simulink model "GNC_functional_diagram"  (R2021b)
settings: Solver=VariableStepAuto  StartTime=0.0  StopTime=10.0  RelTol=1e-3
model workspace (MAT data in the model file):
  AV_Status_Signal = Simulink.Bus
  AV_Status_Signal.Alignment = -1
  AV_Status_Signal.PreserveElementDimensions = 0
  AV_Status_Signal.Elements_internal(1) = Simulink.BusElement
  AV_Status_Signal.Elements_internal(1).DimensionsMode = 'Fixed'
  AV_Status_Signal.Elements_internal(1).SamplingMode = 'Sample based'
  AV_Status_Signal.Elements_internal(1).SampleTime = -1
  AV_Status_Signal.Elements_internal(1).Name = 'Detumbling_Trigger'
  AV_Status_Signal.Elements_internal(1).DataType_internal = 'double'
  AV_Status_Signal.Elements_internal(1).Complexity = 'real'
  AV_Status_Signal.Elements_internal(1).Dimensions = 1
  AV_Status_Signal.Elements_internal(2) = Simulink.BusElement
  AV_Status_Signal.Elements_internal(2).DimensionsMode = 'Fixed'
  AV_Status_Signal.Elements_internal(2).SamplingMode = 'Sample based'
  AV_Status_Signal.Elements_internal(2).SampleTime = -1
  AV_Status_Signal.Elements_internal(2).Name = 'Testing_Trigger'
  AV_Status_Signal.Elements_internal(2).DataType_internal = 'double'
  AV_Status_Signal.Elements_internal(2).Complexity = 'real'
  AV_Status_Signal.Elements_internal(2).Dimensions = 1
  AV_Status_Signal.DataScope = 'Auto'
  Resources_Budget = Simulink.Bus
  Resources_Budget.Alignment = -1
  Resources_Budget.PreserveElementDimensions = 0
  Resources_Budget.Elements_internal(1) = Simulink.BusElement
  Resources_Budget.Elements_internal(1).DimensionsMode = 'Fixed'
  Resources_Budget.Elements_internal(1).SamplingMode = 'Sample based'
  Resources_Budget.Elements_internal(1).SampleTime = -1
  Resources_Budget.Elements_internal(1).Name = 'Processing_Power'
  Resources_Budget.Elements_internal(1).DataType_internal = 'double'
  Resources_Budget.Elements_internal(1).Complexity = 'real'
  Resources_Budget.Elements_internal(1).Dimensions = 1
  Resources_Budget.Elements_internal(2) = Simulink.BusElement
  Resources_Budget.Elements_internal(2).DimensionsMode = 'Fixed'
  Resources_Budget.Elements_internal(2).SamplingMode = 'Sample based'
  Resources_Budget.Elements_internal(2).SampleTime = -1
  Resources_Budget.Elements_internal(2).Name = 'Memory_Allocation'
  Resources_Budget.Elements_internal(2).DataType_internal = 'double'
  Resources_Budget.Elements_internal(2).Complexity = 'real'
  Resources_Budget.Elements_internal(2).Dimensions = 1
  Resources_Budget.Elements_internal(3) = Simulink.BusElement
  Resources_Budget.Elements_internal(3).DimensionsMode = 'Fixed'
  Resources_Budget.Elements_internal(3).SamplingMode = 'Sample based'
  Resources_Budget.Elements_internal(3).SampleTime = -1
  Resources_Budget.Elements_internal(3).Name = 'Power'
  Resources_Budget.Elements_internal(3).DataType_internal = 'double'
  Resources_Budget.Elements_internal(3).Complexity = 'real'
  Resources_Budget.Elements_internal(3).Dimensions = 1
  Resources_Budget.DataScope = 'Auto'
  Sensor_Signal = Simulink.Bus
  Sensor_Signal.Alignment = -1
  Sensor_Signal.PreserveElementDimensions = 0
  Sensor_Signal.Elements_internal(1) = Simulink.BusElement
  Sensor_Signal.Elements_internal(1).DimensionsMode = 'Fixed'
  Sensor_Signal.Elements_internal(1).SamplingMode = 'Sample based'
  Sensor_Signal.Elements_internal(1).SampleTime = -1
  Sensor_Signal.Elements_internal(1).Name = 'Sun_Sensor_Measurment'
  Sensor_Signal.Elements_internal(1).DataType_internal = 'double'
  Sensor_Signal.Elements_internal(1).Complexity = 'real'
  Sensor_Signal.Elements_internal(1).Dimensions = 1
  Sensor_Signal.Elements_internal(2) = Simulink.BusElement
  Sensor_Signal.Elements_internal(2).DimensionsMode = 'Fixed'
  Sensor_Signal.Elements_internal(2).SamplingMode = 'Sample based'
  Sensor_Signal.Elements_internal(2).SampleTime = -1
  Sensor_Signal.Elements_internal(2).Name = 'IMU_Measurement'
  Sensor_Signal.Elements_internal(2).DataType_internal = 'double'
  Sensor_Signal.Elements_internal(2).Complexity = 'real'
  Sensor_Signal.Elements_internal(2).Dimensions = 1
  Sensor_Signal.DataScope = 'Auto'
settings Model: Creator=jonas  LastModifiedBy=leoba

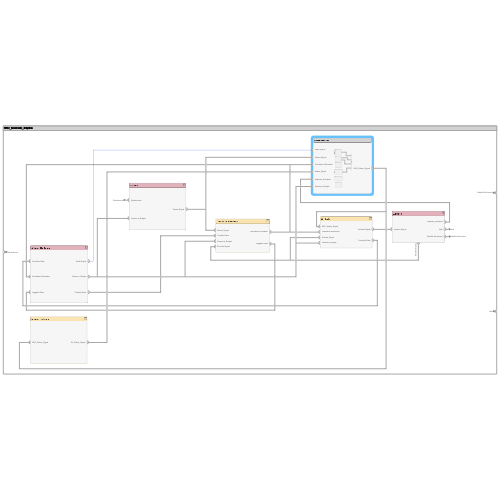
[thumbnail: Simulink's stored preview of the top-level diagram]
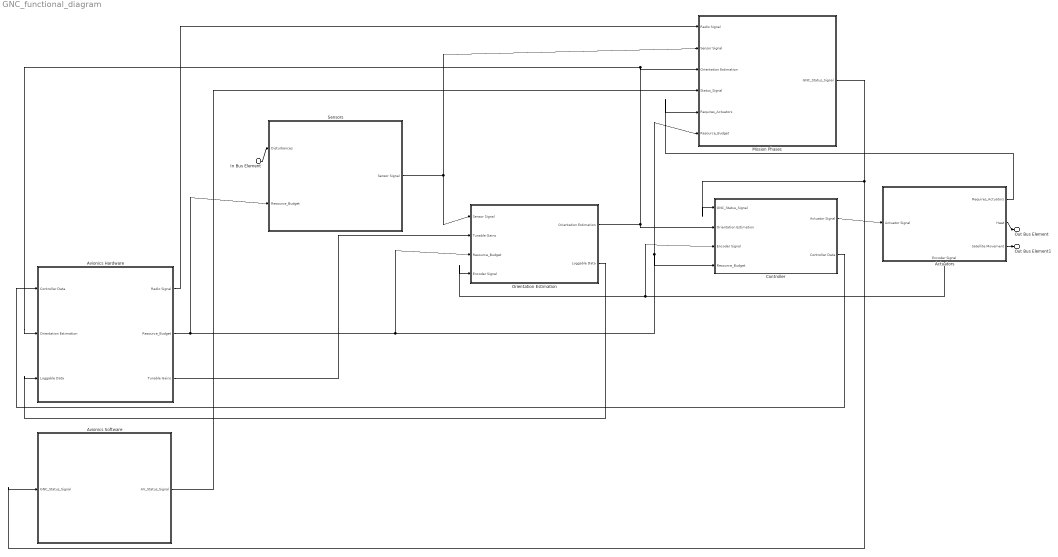
== system GNC_functional_diagram ==
  In Bus Element : Inport  PortName=Disturbances
  Actuators : Subsystem
      settings: PortSchema="{\"entries\":[{\"content\":{\"headerSize\":26,\"margin\":15,\"minimumSpacing\":25,\"sides\":[{\"content\":{\"connectorIds\":[\"In1\"]},\"type\":\"ConnectorPlacement.EquallySpacedRectSide\",\"uuid\":\"4d219d8c-999e-4fa6-ade9-cc6ac14ded32\"},{\"content\":{\"connectorIds\":[\"Out1\",\"Out2\",\"Out3\"],\"side\":\"RIGHT\"},\"type\":\"ConnectorPlacement.EquallySpacedRectSide\",\"uuid\":\"291554bf-cd30-4ae6-93e5-4052e0d4037d\"},{\"content\":{\"connectorIds\":[],\"side\":\"TOP\"},\"type\":\"ConnectorPlacement.EquallySpacedRectSide\",\"uuid\":\"a407b5ba-b8ce-49a8-af7c-64b4689399b6\"},{\"content\":{\"connectorIds\":[\"Out4\"],\"side\":\"BOTTOM\"},\"type\":\"ConnectorPlacement.EquallySpacedRectSide\",\"uuid\":\"28acc806-9e86-4bc6-af71-2b4411156648\"}]},\"type\":\"ConnectorPlacement.EquallySpacedConnector\",\"uuid\":\"1a65b071-c199-4364-8343-b80f4df9252b\"}],\"packageUris\":[\"http://schema.mathworks.com/mf0/Connector/R2020b\"],\"version\":\"1.0\"}"
  Avionics Hardware : Subsystem
      settings: PortSchema="{\"entries\":[{\"content\":{\"headerSize\":26,\"margin\":15,\"minimumSpacing\":25,\"sides\":[{\"content\":{\"connectorIds\":[\"In1\",\"In3\",\"In2\"]},\"type\":\"ConnectorPlacement.EquallySpacedRectSide\",\"uuid\":\"4d219d8c-999e-4fa6-ade9-cc6ac14ded32\"},{\"content\":{\"connectorIds\":[\"Out1\",\"Out2\",\"Out3\"],\"side\":\"RIGHT\"},\"type\":\"ConnectorPlacement.EquallySpacedRectSide\",\"uuid\":\"291554bf-cd30-4ae6-93e5-4052e0d4037d\"},{\"content\":{\"connectorIds\":[],\"side\":\"TOP\"},\"type\":\"ConnectorPlacement.EquallySpacedRectSide\",\"uuid\":\"a407b5ba-b8ce-49a8-af7c-64b4689399b6\"},{\"content\":{\"connectorIds\":[],\"side\":\"BOTTOM\"},\"type\":\"ConnectorPlacement.EquallySpacedRectSide\",\"uuid\":\"eed5de48-d554-4a4a-aaed-8ac1beb8b61e\"}]},\"type\":\"ConnectorPlacement.EquallySpacedConnector\",\"uuid\":\"1a65b071-c199-4364-8343-b80f4df9252b\"}],\"packageUris\":[\"http://schema.mathworks.com/mf0/Connector/R2020b\"],\"version\":\"1.0\"}"
  Avionics Software : Subsystem
      settings: PortSchema="{\"entries\":[{\"content\":{\"headerSize\":26,\"margin\":15,\"minimumSpacing\":25,\"sides\":[{\"content\":{\"connectorIds\":[\"In1\"]},\"type\":\"ConnectorPlacement.EquallySpacedRectSide\",\"uuid\":\"9c9f921c-2c3b-482c-ae0a-30fa5cf19172\"},{\"content\":{\"connectorIds\":[\"Out1\"],\"side\":\"RIGHT\"},\"type\":\"ConnectorPlacement.EquallySpacedRectSide\",\"uuid\":\"566c4868-5865-4e1f-981e-d74a35c979c9\"},{\"content\":{\"connectorIds\":[],\"side\":\"TOP\"},\"type\":\"ConnectorPlacement.EquallySpacedRectSide\",\"uuid\":\"2cd88ae2-a2e5-4e25-b817-9d229c73c4c9\"}]},\"type\":\"ConnectorPlacement.EquallySpacedConnector\",\"uuid\":\"48eadbd9-1de4-4fec-af56-45dc4412e923\"}],\"packageUris\":[\"http://schema.mathworks.com/mf0/Connector/R2020b\"],\"version\":\"1.0\"}"
  Controller : Subsystem
      settings: PortSchema="{\"entries\":[{\"content\":{\"headerSize\":26,\"margin\":15,\"minimumSpacing\":25,\"sides\":[{\"content\":{\"connectorIds\":[\"In1\",\"In2\",\"In3\",\"In4\"]},\"type\":\"ConnectorPlacement.EquallySpacedRectSide\",\"uuid\":\"4d219d8c-999e-4fa6-ade9-cc6ac14ded32\"},{\"content\":{\"connectorIds\":[\"Out1\",\"Out2\"],\"side\":\"RIGHT\"},\"type\":\"ConnectorPlacement.EquallySpacedRectSide\",\"uuid\":\"291554bf-cd30-4ae6-93e5-4052e0d4037d\"},{\"content\":{\"connectorIds\":[],\"side\":\"TOP\"},\"type\":\"ConnectorPlacement.EquallySpacedRectSide\",\"uuid\":\"a407b5ba-b8ce-49a8-af7c-64b4689399b6\"}]},\"type\":\"ConnectorPlacement.EquallySpacedConnector\",\"uuid\":\"1a65b071-c199-4364-8343-b80f4df9252b\"}],\"packageUris\":[\"http://schema.mathworks.com/mf0/Connector/R2020b\"],\"version\":\"1.0\"}"
  Mission Phases : Subsystem
      settings: PortSchema="{\"entries\":[{\"content\":{\"headerSize\":26,\"margin\":15,\"minimumSpacing\":25,\"sides\":[{\"content\":{\"connectorIds\":[\"In1\",\"In2\",\"In3\",\"In4\",\"In5\",\"In6\"]},\"type\":\"ConnectorPlacement.EquallySpacedRectSide\",\"uuid\":\"9c9f921c-2c3b-482c-ae0a-30fa5cf19172\"},{\"content\":{\"connectorIds\":[\"Out1\"],\"side\":\"RIGHT\"},\"type\":\"ConnectorPlacement.EquallySpacedRectSide\",\"uuid\":\"566c4868-5865-4e1f-981e-d74a35c979c9\"},{\"content\":{\"connectorIds\":[],\"side\":\"TOP\"},\"type\":\"ConnectorPlacement.EquallySpacedRectSide\",\"uuid\":\"2cd88ae2-a2e5-4e25-b817-9d229c73c4c9\"}]},\"type\":\"ConnectorPlacement.EquallySpacedConnector\",\"uuid\":\"48eadbd9-1de4-4fec-af56-45dc4412e923\"}],\"packageUris\":[\"http://schema.mathworks.com/mf0/Connector/R2020b\"],\"version\":\"1.0\"}"
  Orientation Estimation : Subsystem
      settings: PortSchema="{\"entries\":[{\"content\":{\"headerSize\":26,\"margin\":15,\"minimumSpacing\":25,\"sides\":[{\"content\":{\"connectorIds\":[\"In1\",\"In2\",\"In3\",\"In4\"]},\"type\":\"ConnectorPlacement.EquallySpacedRectSide\",\"uuid\":\"4d219d8c-999e-4fa6-ade9-cc6ac14ded32\"},{\"content\":{\"connectorIds\":[\"Out1\",\"Out2\"],\"side\":\"RIGHT\"},\"type\":\"ConnectorPlacement.EquallySpacedRectSide\",\"uuid\":\"291554bf-cd30-4ae6-93e5-4052e0d4037d\"},{\"content\":{\"connectorIds\":[],\"side\":\"TOP\"},\"type\":\"ConnectorPlacement.EquallySpacedRectSide\",\"uuid\":\"a407b5ba-b8ce-49a8-af7c-64b4689399b6\"}]},\"type\":\"ConnectorPlacement.EquallySpacedConnector\",\"uuid\":\"1a65b071-c199-4364-8343-b80f4df9252b\"}],\"packageUris\":[\"http://schema.mathworks.com/mf0/Connector/R2020b\"],\"version\":\"1.0\"}"
  Sensors : Subsystem
      settings: PortSchema="{\"entries\":[{\"content\":{\"headerSize\":26,\"margin\":15,\"minimumSpacing\":25,\"sides\":[{\"content\":{\"connectorIds\":[\"In1\",\"In2\"]},\"type\":\"ConnectorPlacement.EquallySpacedRectSide\",\"uuid\":\"4d219d8c-999e-4fa6-ade9-cc6ac14ded32\"},{\"content\":{\"connectorIds\":[\"Out1\"],\"side\":\"RIGHT\"},\"type\":\"ConnectorPlacement.EquallySpacedRectSide\",\"uuid\":\"291554bf-cd30-4ae6-93e5-4052e0d4037d\"},{\"content\":{\"connectorIds\":[],\"side\":\"TOP\"},\"type\":\"ConnectorPlacement.EquallySpacedRectSide\",\"uuid\":\"a407b5ba-b8ce-49a8-af7c-64b4689399b6\"}]},\"type\":\"ConnectorPlacement.EquallySpacedConnector\",\"uuid\":\"1a65b071-c199-4364-8343-b80f4df9252b\"}],\"packageUris\":[\"http://schema.mathworks.com/mf0/Connector/R2020b\"],\"version\":\"1.0\"}"
  Out Bus Element1 : Outport  PortName=Satellite Movement
  Out Bus Element : Outport  Port=2  PortName=Heat
  wires:
  Orientation Estimation/1(Orientation Estimation) -> Avionics Hardware/3(Orientation Estimation), Mission Phases/3(Orientation Estimation), Controller/2(Orientation Estimation)
  Orientation Estimation/2(Loggable Data) -> Avionics Hardware/2(Loggable Data)
  Avionics Hardware/3(Tunable Gains) -> Orientation Estimation/2(Tunable Gains)
  Controller/1(Actuator Signal) -> Actuators/1(Actuator Signal)
  Controller/2(Controller Data) -> Avionics Hardware/1(Controller Data)
  Actuators/4(Encoder Signal) -> Orientation Estimation/4(Encoder Signal), Controller/3(Encoder Signal)
  Actuators/2(Heat) -> Out Bus Element/1
  Actuators/3(Satellite Movement) -> Out Bus Element1/1
  In Bus Element/1 -> Sensors/1(Disturbances)
  Avionics Hardware/1(Radio Signal) -> Mission Phases/1(Radio Signal)
  Sensors/1(Sensor Signal) -> Mission Phases/2(Sensor Signal), Orientation Estimation/1(Sensor Signal)
  Avionics Software/1(AV_Status_Signal) -> Mission Phases/4(Status_Signal)
  Actuators/1(Requires_Actuators) -> Mission Phases/5(Requires_Actuators)
  Mission Phases/1(GNC_Status_Signal) -> Controller/1(GNC_Status_Signal), Avionics Software/1(GNC_Status_Signal)
  Avionics Hardware/2(Resource_Budget) -> Sensors/2(Resource_Budget), Controller/4(Resource_Budget), Mission Phases/6(Resource_Budget), Orientation Estimation/3(Resource_Budget)

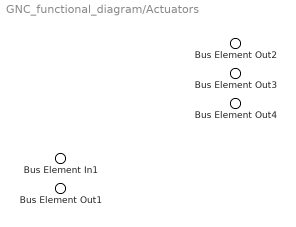
== system GNC_functional_diagram/Actuators ==
  Bus Element In1 : Inport  PortName=Actuator Signal
  Bus Element Out4 : Outport  PortName=Requires_Actuators
  Bus Element Out2 : Outport  Port=2  PortName=Heat
  Bus Element Out3 : Outport  Port=3  PortName=Satellite Movement
  Bus Element Out1 : Outport  Port=4  PortName=Encoder Signal

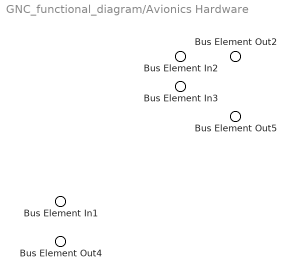
== system GNC_functional_diagram/Avionics Hardware ==
  Bus Element In3 : Inport  PortName=Controller Data
  Bus Element In2 : Inport  Port=2  PortName=Loggable Data
  Bus Element In1 : Inport  Port=3  PortName=Orientation Estimation
  Bus Element Out5 : Outport  PortName=Radio Signal
  Bus Element Out2 : Outport  Port=2  PortName=Resource_Budget
  Bus Element Out4 : Outport  Port=3  PortName=Tunable Gains

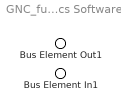
== system GNC_functional_diagram/Avionics Software ==
  Bus Element In1 : Inport  PortName=GNC_Status_Signal
  Bus Element Out1 : Outport  PortName=AV_Status_Signal

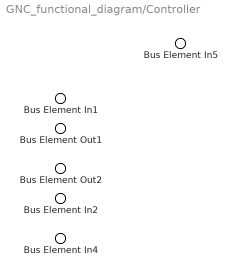
== system GNC_functional_diagram/Controller ==
  Bus Element In5 : Inport  PortName=GNC_Status_Signal
  Bus Element In1 : Inport  Port=2  PortName=Orientation Estimation
  Bus Element In2 : Inport  Port=3  PortName=Encoder Signal
  Bus Element In4 : Inport  Port=4  PortName=Resource_Budget
  Bus Element Out1 : Outport  PortName=Actuator Signal
  Bus Element Out2 : Outport  Port=2  PortName=Controller Data

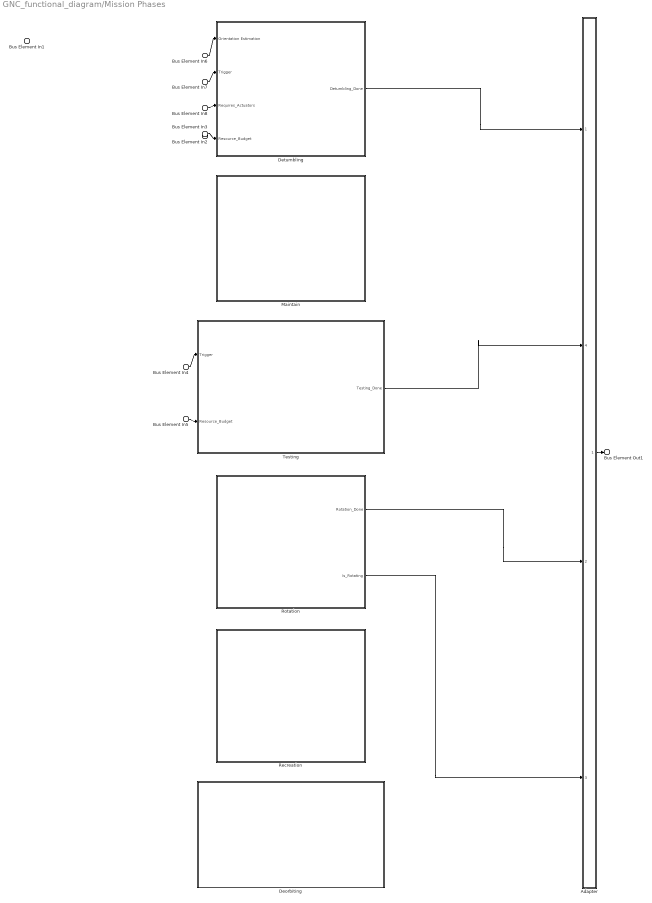
== system GNC_functional_diagram/Mission Phases ==
  Bus Element In1 : Inport  PortName=Radio Signal
  Bus Element In2 : Inport  Port=2  PortName=Sensor Signal
  Bus Element In6 : Inport  Port=3  PortName=Orientation Estimation
  Bus Element In7 : Inport  Port=4  PortName=Status_Signal  Element=Detumbling_Trigger
  Bus Element In4 : Inport  Port=4  PortName=Status_Signal  Element=Testing_Trigger
  Bus Element In8 : Inport  Port=5  PortName=Requires_Actuators
  Bus Element In3 : Inport  Port=6  PortName=Resource_Budget
  Bus Element In5 : Inport  Port=6  PortName=Resource_Budget
  Adapter : Subsystem
      settings: PortSchema="{\"entries\":[{\"content\":{\"margin\":10,\"minimumSpacing\":15,\"sides\":[{\"content\":{\"connectorIds\":[\"In1\",\"In4\",\"In2\",\"In3\"]},\"type\":\"ConnectorPlacement.EquallySpacedRectSide\",\"uuid\":\"9c9f921c-2c3b-482c-ae0a-30fa5cf19172\"},{\"content\":{\"connectorIds\":[\"Out1\"],\"side\":\"RIGHT\"},\"type\":\"ConnectorPlacement.EquallySpacedRectSide\",\"uuid\":\"566c4868-5865-4e1f-981e-d74a35c979c9\"},{\"content\":{\"connectorIds\":[],\"side\":\"TOP\"},\"type\":\"ConnectorPlacement.EquallySpacedRectSide\",\"uuid\":\"2cd88ae2-a2e5-4e25-b817-9d229c73c4c9\"}]},\"type\":\"ConnectorPlacement.EquallySpacedConnector\",\"uuid\":\"48eadbd9-1de4-4fec-af56-45dc4412e923\"}],\"packageUris\":[\"http://schema.mathworks.com/mf0/Connector/R2020b\"],\"version\":\"1.0\"}"
  Deorbiting : Subsystem
      settings: PortSchema="{\"entries\":[{\"content\":{\"headerSize\":26,\"margin\":15,\"minimumSpacing\":25,\"sides\":[{\"content\":{\"connectorIds\":[]},\"type\":\"ConnectorPlacement.EquallySpacedRectSide\",\"uuid\":\"9c9f921c-2c3b-482c-ae0a-30fa5cf19172\"},{\"content\":{\"connectorIds\":[],\"side\":\"RIGHT\"},\"type\":\"ConnectorPlacement.EquallySpacedRectSide\",\"uuid\":\"566c4868-5865-4e1f-981e-d74a35c979c9\"},{\"content\":{\"connectorIds\":[],\"side\":\"TOP\"},\"type\":\"ConnectorPlacement.EquallySpacedRectSide\",\"uuid\":\"2cd88ae2-a2e5-4e25-b817-9d229c73c4c9\"}]},\"type\":\"ConnectorPlacement.EquallySpacedConnector\",\"uuid\":\"48eadbd9-1de4-4fec-af56-45dc4412e923\"}],\"packageUris\":[\"http://schema.mathworks.com/mf0/Connector/R2020b\"],\"version\":\"1.0\"}"
  Detumbling : Subsystem
      settings: PortSchema="{\"entries\":[{\"content\":{\"headerSize\":26,\"margin\":15,\"minimumSpacing\":25,\"sides\":[{\"content\":{\"connectorIds\":[\"In1\",\"In2\",\"In3\",\"In4\"]},\"type\":\"ConnectorPlacement.EquallySpacedRectSide\",\"uuid\":\"9c9f921c-2c3b-482c-ae0a-30fa5cf19172\"},{\"content\":{\"connectorIds\":[\"Out1\"],\"side\":\"RIGHT\"},\"type\":\"ConnectorPlacement.EquallySpacedRectSide\",\"uuid\":\"566c4868-5865-4e1f-981e-d74a35c979c9\"},{\"content\":{\"connectorIds\":[],\"side\":\"TOP\"},\"type\":\"ConnectorPlacement.EquallySpacedRectSide\",\"uuid\":\"2cd88ae2-a2e5-4e25-b817-9d229c73c4c9\"}]},\"type\":\"ConnectorPlacement.EquallySpacedConnector\",\"uuid\":\"48eadbd9-1de4-4fec-af56-45dc4412e923\"}],\"packageUris\":[\"http://schema.mathworks.com/mf0/Connector/R2020b\"],\"version\":\"1.0\"}"
  Maintain : Subsystem
      settings: PortSchema="{\"entries\":[{\"content\":{\"headerSize\":26,\"margin\":15,\"minimumSpacing\":25,\"sides\":[{\"content\":{\"connectorIds\":[]},\"type\":\"ConnectorPlacement.EquallySpacedRectSide\",\"uuid\":\"9c9f921c-2c3b-482c-ae0a-30fa5cf19172\"},{\"content\":{\"connectorIds\":[],\"side\":\"RIGHT\"},\"type\":\"ConnectorPlacement.EquallySpacedRectSide\",\"uuid\":\"566c4868-5865-4e1f-981e-d74a35c979c9\"},{\"content\":{\"connectorIds\":[],\"side\":\"TOP\"},\"type\":\"ConnectorPlacement.EquallySpacedRectSide\",\"uuid\":\"2cd88ae2-a2e5-4e25-b817-9d229c73c4c9\"}]},\"type\":\"ConnectorPlacement.EquallySpacedConnector\",\"uuid\":\"48eadbd9-1de4-4fec-af56-45dc4412e923\"}],\"packageUris\":[\"http://schema.mathworks.com/mf0/Connector/R2020b\"],\"version\":\"1.0\"}"
  Recreation : Subsystem
      settings: PortSchema="{\"entries\":[{\"content\":{\"headerSize\":26,\"margin\":15,\"minimumSpacing\":25,\"sides\":[{\"content\":{\"connectorIds\":[]},\"type\":\"ConnectorPlacement.EquallySpacedRectSide\",\"uuid\":\"9c9f921c-2c3b-482c-ae0a-30fa5cf19172\"},{\"content\":{\"connectorIds\":[],\"side\":\"RIGHT\"},\"type\":\"ConnectorPlacement.EquallySpacedRectSide\",\"uuid\":\"566c4868-5865-4e1f-981e-d74a35c979c9\"},{\"content\":{\"connectorIds\":[],\"side\":\"TOP\"},\"type\":\"ConnectorPlacement.EquallySpacedRectSide\",\"uuid\":\"2cd88ae2-a2e5-4e25-b817-9d229c73c4c9\"}]},\"type\":\"ConnectorPlacement.EquallySpacedConnector\",\"uuid\":\"48eadbd9-1de4-4fec-af56-45dc4412e923\"}],\"packageUris\":[\"http://schema.mathworks.com/mf0/Connector/R2020b\"],\"version\":\"1.0\"}"
  Rotation : Subsystem
      settings: PortSchema="{\"entries\":[{\"content\":{\"headerSize\":26,\"margin\":15,\"minimumSpacing\":25,\"sides\":[{\"content\":{\"connectorIds\":[]},\"type\":\"ConnectorPlacement.EquallySpacedRectSide\",\"uuid\":\"9c9f921c-2c3b-482c-ae0a-30fa5cf19172\"},{\"content\":{\"connectorIds\":[\"Out1\",\"Out2\"],\"side\":\"RIGHT\"},\"type\":\"ConnectorPlacement.EquallySpacedRectSide\",\"uuid\":\"566c4868-5865-4e1f-981e-d74a35c979c9\"},{\"content\":{\"connectorIds\":[],\"side\":\"TOP\"},\"type\":\"ConnectorPlacement.EquallySpacedRectSide\",\"uuid\":\"2cd88ae2-a2e5-4e25-b817-9d229c73c4c9\"}]},\"type\":\"ConnectorPlacement.EquallySpacedConnector\",\"uuid\":\"48eadbd9-1de4-4fec-af56-45dc4412e923\"}],\"packageUris\":[\"http://schema.mathworks.com/mf0/Connector/R2020b\"],\"version\":\"1.0\"}"
  Testing : Subsystem
      settings: PortSchema="{\"entries\":[{\"content\":{\"headerSize\":26,\"margin\":15,\"minimumSpacing\":25,\"sides\":[{\"content\":{\"connectorIds\":[\"In1\",\"In2\"]},\"type\":\"ConnectorPlacement.EquallySpacedRectSide\",\"uuid\":\"9c9f921c-2c3b-482c-ae0a-30fa5cf19172\"},{\"content\":{\"connectorIds\":[\"Out1\"],\"side\":\"RIGHT\"},\"type\":\"ConnectorPlacement.EquallySpacedRectSide\",\"uuid\":\"566c4868-5865-4e1f-981e-d74a35c979c9\"},{\"content\":{\"connectorIds\":[],\"side\":\"TOP\"},\"type\":\"ConnectorPlacement.EquallySpacedRectSide\",\"uuid\":\"2cd88ae2-a2e5-4e25-b817-9d229c73c4c9\"}]},\"type\":\"ConnectorPlacement.EquallySpacedConnector\",\"uuid\":\"48eadbd9-1de4-4fec-af56-45dc4412e923\"}],\"packageUris\":[\"http://schema.mathworks.com/mf0/Connector/R2020b\"],\"version\":\"1.0\"}"
  Bus Element Out1 : Outport  PortName=GNC_Status_Signal
  wires:
  Bus Element In6/1 -> Detumbling/1(Orientation Estimation)
  Bus Element In7/1 -> Detumbling/2(Trigger)
  Bus Element In8/1 -> Detumbling/3(Requires_Actuators)
  Detumbling/1(Detumbling_Done) -> Adapter/1(Detumbling_Done)
  Rotation/1(Rotation_Done) -> Adapter/2(Rotation_Done)
  Rotation/2(Is_Rotating) -> Adapter/3(Is_Rotating)
  Adapter/1(GNC_Status_) -> Bus Element Out1/1
  Bus Element In3/1 -> Detumbling/4(Resource_Budget)
  Testing/1(Testing_Done) -> Adapter/4(Testing_Done)
  Bus Element In4/1 -> Testing/1(Trigger)
  Bus Element In5/1 -> Testing/2(Resource_Budget)

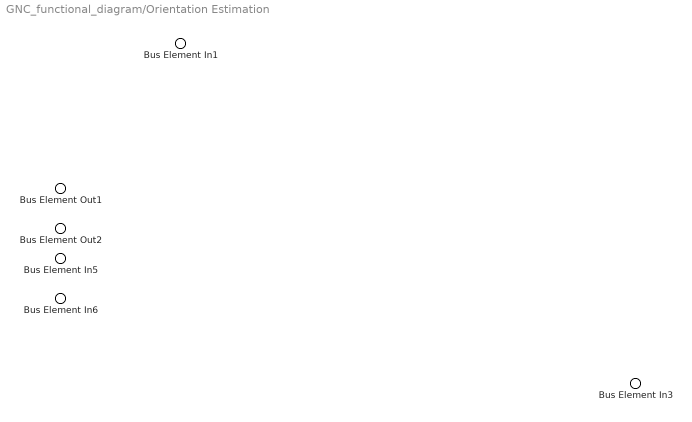
== system GNC_functional_diagram/Orientation Estimation ==
  Bus Element In3 : Inport  PortName=Sensor Signal  Element=IMU_Measurement
  Bus Element In5 : Inport  Port=2  PortName=Tunable Gains
  Bus Element In1 : Inport  Port=3  PortName=Resource_Budget
  Bus Element In6 : Inport  Port=4  PortName=Encoder Signal
  Bus Element Out1 : Outport  PortName=Orientation Estimation
  Bus Element Out2 : Outport  Port=2  PortName=Loggable Data

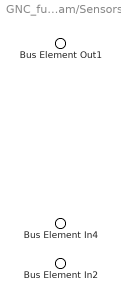
== system GNC_functional_diagram/Sensors ==
  Bus Element In4 : Inport  PortName=Disturbances
  Bus Element In2 : Inport  Port=2  PortName=Resource_Budget
  Bus Element Out1 : Outport  PortName=Sensor Signal

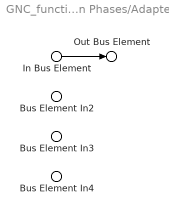
== system GNC_functional_diagram/Mission Phases/Adapter ==
  In Bus Element : Inport  PortName=Detumbling_Done
  Bus Element In2 : Inport  Port=2  PortName=Rotation_Done
  Bus Element In3 : Inport  Port=3  PortName=Is_Rotating
  Bus Element In4 : Inport  Port=4  PortName=Testing_Done
  Out Bus Element : Outport  PortName=GNC_Status_
  wires:
  In Bus Element/1 -> Out Bus Element/1

== system GNC_functional_diagram/Mission Phases/Deorbiting ==

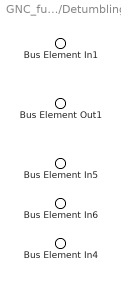
== system GNC_functional_diagram/Mission Phases/Detumbling ==
  Bus Element In1 : Inport  PortName=Orientation Estimation
  Bus Element In5 : Inport  Port=2  PortName=Trigger
  Bus Element In6 : Inport  Port=3  PortName=Requires_Actuators
  Bus Element In4 : Inport  Port=4  PortName=Resource_Budget
  Bus Element Out1 : Outport  PortName=Detumbling_Done

== system GNC_functional_diagram/Mission Phases/Maintain ==

== system GNC_functional_diagram/Mission Phases/Recreation ==

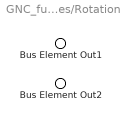
== system GNC_functional_diagram/Mission Phases/Rotation ==
  Bus Element Out1 : Outport  PortName=Rotation_Done
  Bus Element Out2 : Outport  Port=2  PortName=Is_Rotating

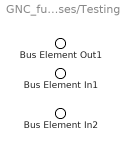
== system GNC_functional_diagram/Mission Phases/Testing ==
  Bus Element In1 : Inport  PortName=Trigger
  Bus Element In2 : Inport  Port=2  PortName=Resource_Budget
  Bus Element Out1 : Outport  PortName=Testing_Done
